simulink model "untitled1"  (R2021b)
settings: Solver=ode4  StartTime=TIME.Start  StopTime=TIME.Final  FixedStep=TIME.Ts  RelTol=1e-3
values from neighbouring files (symbols this model uses):
  bias = -3.0    (= -3)    [main_untitled1.m]    (also in main_untitled2.m = 1.5)
  den = [1 2*sqrt(3)*sqrt(2) 3]    [main_simulink_practice.m]    (also in main_untitled1.m = [1 2*zt*Wn Wn^2]; main_untitled2.m = [1 0])
  mag = 2.0    (= 2)    [main_simulink_practice.m]    (also in main_untitled1.m = 1.5; main_untitled2.m = 1.5)
  num = 3    [main_simulink_practice.m]    (also in main_untitled1.m = 144; main_untitled2.m = 1)
  omega = 2*pi*freq    (= 3.14159265359)    [main_untitled1.m]    (also in main_untitled2.m; script_simulation2.m = 10^N)
  phs = 20*pi/180.0    (= 0.349065850399)    [main_simulink_practice.m]    (also in main_untitled1.m = 0.261799387799; main_untitled2.m = deg2rad(15))
  TIME = struct('Ts'   , 1e-3,                'Start', 0.0 ,                'Final',20.0 ,                'stage', 0.15,                'time' , 0   ,                'Ntime', 0   )    [UAV_simulation.m]    (also in main_simulink_practice.m = struct('Start', 0.0,                'Ts'   , 1e-3,          ; main_untitled1.m = struct('Ts', 1e-3,                'Final',30,               ; main_untitled2.m = struct('Ts', 1e-3,                'Start', 0.0,             ; script_simulation.m = struct('Start', 0.0  ,                'Final',30.0  ,       )
settings Model: Creator=jinkwak  LastModifiedBy=jinkwak

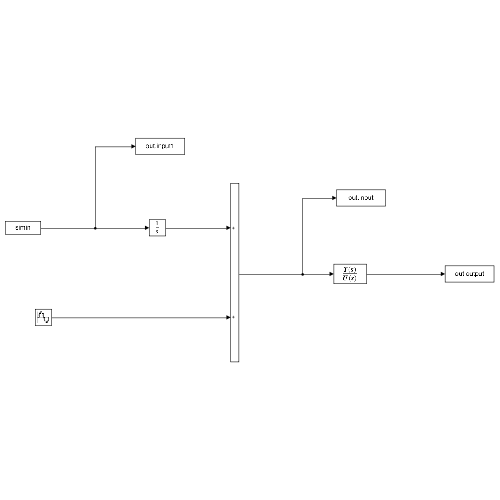
[thumbnail: Simulink's stored preview of the top-level diagram]
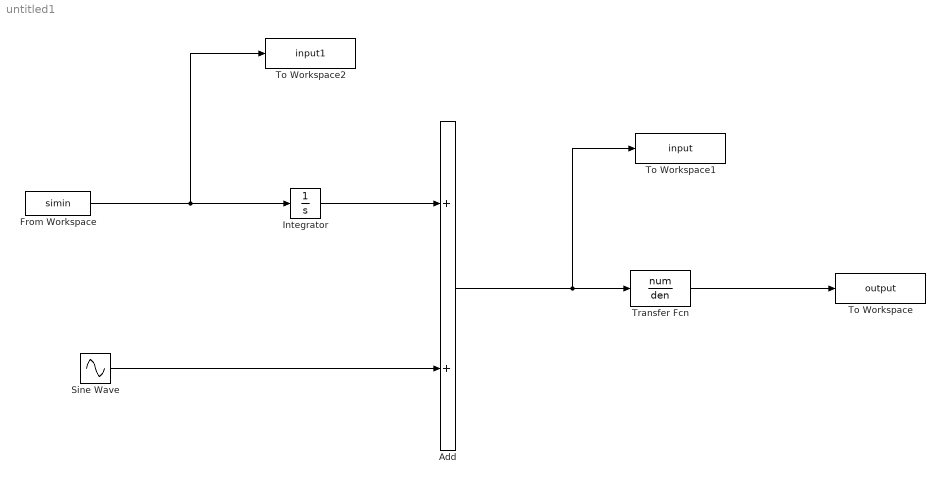
== system untitled1 ==
  Add : Sum
  From Workspace : FromWorkspace  VariableName=simin  SampleTime=TIME.Ts
  Integrator : Integrator
  Sine Wave : Sin  Amplitude=mag  Bias=bias  Frequency=omega  Phase=phs  SampleTime=TIME.Ts
  To Workspace : ToWorkspace  VariableName=output  SampleTime=TIME.Ts
      settings: Save2DSignal=2-D array (concatenate along first dimension)
  To Workspace1 : ToWorkspace  VariableName=input  SampleTime=TIME.Ts
      settings: Save2DSignal=2-D array (concatenate along first dimension)
  To Workspace2 : ToWorkspace  VariableName=input1  SampleTime=TIME.Ts
      settings: Save2DSignal=2-D array (concatenate along first dimension)
  Transfer Fcn : TransferFcn  Numerator=num  Denominator=den
  wires:
  Sine Wave/1 -> Add/2
  Integrator/1 -> Add/1
  From Workspace/1 -> To Workspace2/1, Integrator/1
  Add/1 -> To Workspace1/1, Transfer Fcn/1
  Transfer Fcn/1 -> To Workspace/1
